simulink model "psbmachinesR12"  (Simulink 4.00)
settings: Solver=ode15s  SolverMode=SingleTasking  StartTime=0.0  StopTime=5  RelTol=1e-3  AbsTol=1e-3
InitFcn:
  | powericon('psbinitsys',bdroot);
undefined symbols (not defined in the file): D1, Delta
libraries: powerlib2 x14, powerlib_extras x5, powerlib11 x2
settings Model: Creator=patrice  LastModifiedBy=pavel  OutputTimes=[0:1/20:10]  LimitDataPoints=off  RTWTemplateMakefile=grt_unix.tmf  ExtModeTrigMode=oneshot  ExtModeArmWhenConnect=off  BlockReductionOpt=off

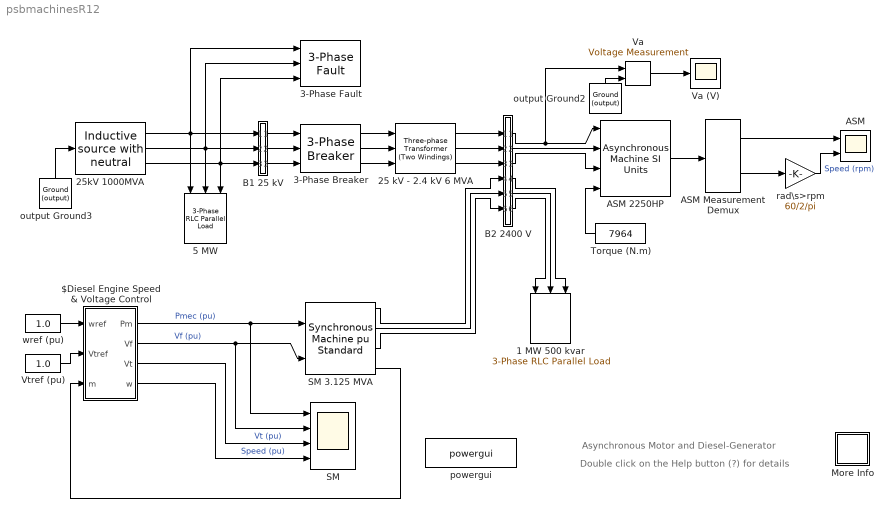
== system psbmachinesR12 ==
  note: Asynchronous Motor and Diesel-Generator
  note: Double click on the Help button (?) for details
  $Diesel Engine Speed & Voltage Control : Subsystem
      settings: RTWFcnNameOpts=Auto  RTWFileNameOpts=Auto
  1 MW 500 kvar : powerlib_extras/Three-Phase Library/3-Phase RLC Parallel Load  Orientation=down  Vpp=2400  fn=60  P3=1e6  QL3=0  QC3=500e3
  25 kV - 2.4 kV 6 MVA : powerlib2/Elements/Three-phase Transformer (Two Windings)  Tag=PoWeRsYsTeMbLoCk  nominal=[ 6e6 , 60 ]  type1=Yg  params1=[ 25e3 , 0.0015 , 0.03]  type2=Delta (D1)  params2=[ 2.4e3 , 0.0015 , 0.03 ]  ynsat=off  rmag=200  lm=200  sat="[ 0,0  ;  0.005,1.2  ;  1.0,1.4 ]"  sif=off  phi0=[ 0.8 , -0.8 , 0.7 ]  mesure=None  PSBOutputType=1111
  25kV 1000MVA : powerlib_extras/Three-Phase Library/Inductive source with neutral  V=25e3/sqrt(3)*sqrt(2)  Phi=0  F=60  R=25^2/1000/10  L=25^2/1000/377
  3-Phase Breaker : powerlib_extras/Three-Phase Library/3-Phase Breaker  init_states=closed  sa=on  sb=on  sc=on  sw_times=[0.2]  Ts=0  comext=off  Ron=0.01  Rp=1e5  Cp=inf  mesure=None
  3-Phase Fault : powerlib_extras/Three-Phase Library/3-Phase Fault  sa=on  sb=on  sc=on  Rdef=0.01  st=on  Rt=0.001  comext=off  sw_status=[1 0]  sw_times=[ 0.1 0.4]  Ts=0  init_statext=[1 1 0]  Rp=inf  Cp=inf  mesure=None
  5 MW : powerlib_extras/Three-Phase Library/3-Phase RLC Parallel Load  Orientation=down  Vpp=25e3  fn=60  P3=5e6  QL3=0  QC3=0
  ASM : Scope  NumInputPorts=2
      settings: TimeRange=0.2  YMin=-7500~1710  YMax=7500~1800  SaveToWorkspace=off  SaveName=ScopeData  DataFormat=Array  MaxDataPoints=5000
  ASM 2250HP : powerlib2/Machines/Asynchronous Machine SI Units  Tag=PoWeRsYsTeMbLoCk  rotType=Squirrel-cage  ctrl=Rotor  x1=[ 2250*746, 2400, 60 ]  x2=[ 0.029 0.226/377]  x3=[ 0.022 0.226/377]  x4=13.04/377  x5="[ 63.87 0  2 ]"  x6=[1 0 0 0 0 0 0 0]  PSBOutputType=1110  iounits=1
  ASM Measurement Demux : powerlib11/Machines/ASM Measurement Demux  a=off  b=off  c=off  d=off  e=on  f=off  g=off  h=off  i=on  j=off  k=off
  B1 25 kV : Subsystem
      settings: RTWFcnNameOpts=Auto  RTWFileNameOpts=Auto
      mask Display: disp('')
  B2 2400 V : Subsystem
      settings: RTWFcnNameOpts=Auto  RTWFileNameOpts=Auto
      mask Display: disp('')
  More Info : Subsystem
      settings: RTWFcnNameOpts=Auto  RTWFileNameOpts=Auto
      mask Display: disp('?')
  SM : Scope  NumInputPorts=4
      settings: TimeRange=0.2  YMin=0.8025~0~0.9825~1.00115  YMax=0.8175~2.75~1.005~1.00155  SaveName=Pmec_SM  DataFormat=Structure  MaxDataPoints=5000  Decimation=10
  SM 3.125 MVA : powerlib2/Machines/Synchronous Machine pu Standard  Tag=PoWeRsYsTeMbLoCk  rotorType=Salient-pole  x1="[ 3.125e6  2400  60 ]"  x2b=[ 31 32 33 34 35 36 37 ]  x2=[ 1.56, 0.296, 0.177, 1.06, 0.177, 0.052 ]  dAxisT=Short-circuit  qAxisT=Open-circuit  x3a=[]  x3b=[]  x3c=[]  x3d=[]  x3=[ 3.7, 0.05, 0.05 ]  x3e=[]  x3f=[]  x3g=[]  x4=0.0036  x5="[ 1.07  0  2 ]"  x6=[0 0 0 0 0 0 0 0 1]  x7=off  x8=[0.211 0.418 1.0 1.72 3.35 ; 0.25 0.50 1.0 1.2 1.4]  PSBOutputType=1110  iounits=0.5
  Torque (N.m) : Constant  Orientation=left  Value=7964
  Va : powerlib2/Measurements/Voltage Measurement  Tag=PoWeRsYsTeMmEaSuReMeNt  PSBOutputType=0  PSBequivalent=0
  Va (V) : Scope
      settings: TickLabels=on  TimeRange=0.2  YMin=-2000  YMax=2000  SaveToWorkspace=off  SaveName=ScopeData  DataFormat=Array  MaxDataPoints=5000
  Vtref (pu) : Constant  Value=1.0
  output Ground2 : powerlib2/Connectors/Ground (output)  Tag=PoWeRsYsTeMbLoCk  Orientation=up  PSBOutputType=1
  output Ground3 : powerlib2/Connectors/Ground (output)  Tag=PoWeRsYsTeMbLoCk  Orientation=up  PSBOutputType=1
  powergui : powerlib2/powergui  matfilesaved=off  Frange=logspace(0,3,50)  Ylog=off  Xlog=off  save=off  variable=ZData  display=off
  rad\s>rpm : Gain  Gain=60/2/pi  Multiplication=Element-wise(K.*u)  SaturateOnIntegerOverflow=on
  wref (pu) : Constant  Value=1.0
  wires:
  25kV 1000MVA/3 -> B1 25 kV/3(C1), 5 MW/3, 3-Phase Fault/3
  25kV 1000MVA/2 -> B1 25 kV/2(B1), 5 MW/2, 3-Phase Fault/2
  25kV 1000MVA/1 -> B1 25 kV/1(A1), 5 MW/1, 3-Phase Fault/1
  output Ground3/1 -> 25kV 1000MVA/1
  B1 25 kV/3(C2) -> 3-Phase Breaker/3
  B1 25 kV/2(B2) -> 3-Phase Breaker/2
  B1 25 kV/1(A2) -> 3-Phase Breaker/1
  3-Phase Breaker/1 -> 25 kV - 2.4 kV 6 MVA/1
  wref (pu)/1 -> $Diesel Engine Speed & Voltage Control/1(wref)
  SM 3.125 MVA/4 -> $Diesel Engine Speed & Voltage Control/3(m)
  Vtref (pu)/1 -> $Diesel Engine Speed & Voltage Control/2(Vtref)
  3-Phase Breaker/3 -> 25 kV - 2.4 kV 6 MVA/3
  3-Phase Breaker/2 -> 25 kV - 2.4 kV 6 MVA/2
  25 kV - 2.4 kV 6 MVA/3 -> B2 2400 V/3(C1)
  25 kV - 2.4 kV 6 MVA/2 -> B2 2400 V/2(B1)
  25 kV - 2.4 kV 6 MVA/1 -> B2 2400 V/1(A1`)
  SM 3.125 MVA/1 -> B2 2400 V/4(A2)
  SM 3.125 MVA/2 -> B2 2400 V/5(B2)
  SM 3.125 MVA/3 -> B2 2400 V/6(C2)
  B2 2400 V/1(A3) -> ASM 2250HP/1, Va/1
  Torque (N.m)/1 -> ASM 2250HP/4
  ASM 2250HP/1 -> ASM Measurement Demux/1
  B2 2400 V/4(A4) -> 1 MW 500 kvar/3
  B2 2400 V/5(B4) -> 1 MW 500 kvar/2
  B2 2400 V/6(C4) -> 1 MW 500 kvar/1
  B2 2400 V/2(B3) -> ASM 2250HP/2
  B2 2400 V/3(C3) -> ASM 2250HP/3
  Va/1 -> Va (V)/1
  output Ground2/1 -> Va/2
  $Diesel Engine Speed & Voltage Control/1(Pm) -> SM 3.125 MVA/1, SM/1  "Pmec (pu)"
  $Diesel Engine Speed & Voltage Control/2(Vf) -> SM 3.125 MVA/2, SM/2  "Vf (pu)"
  $Diesel Engine Speed & Voltage Control/3(Vt) -> SM/3  "Vt (pu)"
  $Diesel Engine Speed & Voltage Control/4(w) -> SM/4  "Speed (pu)"
  ASM Measurement Demux/2 -> rad\s>rpm/1
  ASM Measurement Demux/1 -> ASM/1
  rad\s>rpm/1 -> ASM/2  "Speed (rpm)"

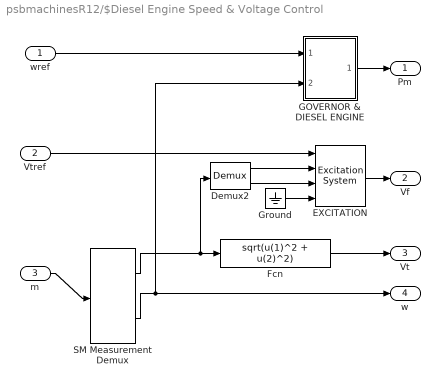
== system psbmachinesR12/$Diesel Engine Speed & Voltage Control ==
  wref : Inport  Port=1
  Vtref : Inport  Port=2
  m : Inport  Port=3
  Demux2 : Demux  Outputs=2  BusSelectionMode=off
  EXCITATION : powerlib2/Machines/Excitation System  tr=20e-3  reg=[ 200, 0.02 ]  exc=[ 1, 0 ]  tgr=[ 0, 0 ]  damp=[ 0.001, 0.1 ]  sat=[ 0, 0 ]  lim=[ 0, 6, 0 ]  v0="[1.0  1.182]"
  Fcn : Fcn  Expr=sqrt(u(1)^2 + u(2)^2)
  GOVERNOR & DIESEL ENGINE : Subsystem  mask(Diesel Engine & Governor){K=40, Tr=[0.01 0.02 0.2], Ta=[0.25 0.009 0.0384], Tlim=[0 1.1], Td=0.024, Pm0=0.1601}
      mask prompts: K "Regulator gain K:"; Tr "Regulator time constants [T1 T2 T3 ] (s) :"; Ta "Actuator time constants [T4 T5 T6] (s) :"; Tlim "Torque limits [Tmin Tmax] (pu) :"; Td "Engine time delay Td (s) :"; Pm0 "Initial value of mechanical power  Pm0 (pu) :"
      mask help:
      | This block implements a diesel engine and governor system:
      | 1st and 2nd inputs: Desired and actual speed (pu)
      | Output: Diesel engine mechanical power.Motor inertia should be combined with generator.
      | Controller transfer function:
      |      Hc=K.(1+T3.s)/(1+T1.s+T1.T2.s^2)
      | Actuator transfer function :
      |      Ha= (1+T4.s) / [ (s (1+T5.s)(1+T6.s) ]
      | Motor :
      |      Time delay Td
      |
      | (See reference in Tutorial Session 5)
      settings: RTWFcnNameOpts=Auto  RTWFileNameOpts=Auto
  Ground : Ground
  SM Measurement Demux : powerlib11/Machines/SM Measurement Demux  a=off  b=off  c=off  d=off  e=off  f=on  g=off  h=on  i=off  j=off
  Pm : Outport  Port=1  InitialOutput=0
  Vf : Outport  Port=2  InitialOutput=0
  Vt : Outport  Port=3  InitialOutput=0
  w : Outport  Port=4  InitialOutput=0
  wires:
  Fcn/1 -> Vt/1
  SM Measurement Demux/1 -> Fcn/1, Demux2/1
  Demux2/1 -> EXCITATION/2
  Vtref/1 -> EXCITATION/1
  GOVERNOR & DIESEL ENGINE/1(Pmec (pu)) -> Pm/1
  EXCITATION/1 -> Vf/1
  Demux2/2 -> EXCITATION/3
  wref/1 -> GOVERNOR & DIESEL ENGINE/1(wref (pu))
  SM Measurement Demux/2 -> w/1, GOVERNOR & DIESEL ENGINE/2(w (pu))
  m/1 -> SM Measurement Demux/1
  Ground/1 -> EXCITATION/4

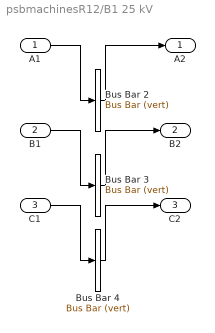
== system psbmachinesR12/B1 25 kV ==
  A1 : Inport  Port=1
  B1 : Inport  Port=2
  C1 : Inport  Port=3
  Bus Bar 2 : powerlib2/Connectors/Bus Bar (vert)  Tag=PoWeRsYsTeMbLoCk  entrees=1  sorties=1  PSBOutputType=11111111111111111111111111111111111111111111111111111111111111111111111111111111111111111
  Bus Bar 3 : powerlib2/Connectors/Bus Bar (vert)  Tag=PoWeRsYsTeMbLoCk  entrees=1  sorties=1  PSBOutputType=11111111111111111111111111111111111111111111111111111111111111111111111111111111111111111
  Bus Bar 4 : powerlib2/Connectors/Bus Bar (vert)  Tag=PoWeRsYsTeMbLoCk  entrees=1  sorties=1  PSBOutputType=11111111111111111111111111111111111111111111111111111111111111111111111111111111111111111
  A2 : Outport  Port=1  InitialOutput=0
  B2 : Outport  Port=2  InitialOutput=0
  C2 : Outport  Port=3  InitialOutput=0
  wires:
  A1/1 -> Bus Bar 2/1
  Bus Bar 2/1 -> A2/1
  B1/1 -> Bus Bar 3/1
  Bus Bar 3/1 -> B2/1
  C1/1 -> Bus Bar 4/1
  Bus Bar 4/1 -> C2/1

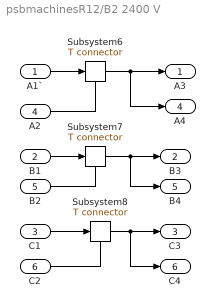
== system psbmachinesR12/B2 2400 V ==
  A1` : Inport  Port=1
  B1 : Inport  Port=2
  C1 : Inport  Port=3
  A2 : Inport  Port=4
  B2 : Inport  Port=5
  C2 : Inport  Port=6
  Subsystem6 : powerlib2/Connectors/T connector  Tag=PoWeRsYsTeMbLoCk  PSBOutputType=1
  Subsystem7 : powerlib2/Connectors/T connector  Tag=PoWeRsYsTeMbLoCk  PSBOutputType=1
  Subsystem8 : powerlib2/Connectors/T connector  Tag=PoWeRsYsTeMbLoCk  PSBOutputType=1
  A3 : Outport  Port=1  InitialOutput=0
  B3 : Outport  Port=2  InitialOutput=0
  C3 : Outport  Port=3  InitialOutput=0
  A4 : Outport  Port=4  InitialOutput=0
  B4 : Outport  Port=5  InitialOutput=0
  C4 : Outport  Port=6  InitialOutput=0
  wires:
  Subsystem8/1 -> C4/1, C3/1
  Subsystem7/1 -> B4/1, B3/1
  Subsystem6/1 -> A4/1, A3/1
  C2/1 -> Subsystem8/Enable
  A2/1 -> Subsystem6/Enable
  B2/1 -> Subsystem7/Enable
  B1/1 -> Subsystem7/1
  C1/1 -> Subsystem8/1
  A1`/1 -> Subsystem6/1

== system psbmachinesR12/More Info ==
  note: Observe that during the fault the terminal voltage drops to about 0.2 pu and the excitation voltage hits the  limit of 6 pu. After fault clearing and islanding
      |  the SM  mechanical power  increases from its initial value of 0.16 pu to the final value of 0.80 pu required by the resistive and motor load (2.49 MW) . After 3 seconds,
      |  the terminal voltage stabilizes at 1 pu. The motor speed decreases transiently from 1789 rpm to 1624 rpm, then it recovers close to its normal value after 2 seconds.
      |
      | If you  increase the fault duration to 12 cycles by changing the breaker opening time to 0.3s, you will notice that the system collapses.
      |  The ASM speed slows down to zero after 2 seconds.
  note: 3
  note: 1
  note: Demonstration
  note: Circuit Description
  note: This demonstration illustrates fault and islanding of an induction motor/diesel-generator system.
      | It also demonstrates the Machine Load Flow option of the PowerGUI .
      | ( See Tutorial Session 5)
  note: A plant consisting of a resistive and motor load (ASM) is fed at 2400 V from a distibution 25 kV network through a 6 MVA 25/2.kV Wye-Delta transformer and from an
      | emergency synchronous generator/ diesel engine unit (SM). The 25 kV network is modelled by a simple R-L equivalent source (short-circuit level 1000 MVA) and a 5 MW load.
      |  The  asynchronous motor is  rated 2250 HP, 2.4 kV and the synchronous machine is rated 3.125 MVA, 2.4kV. The SM excitation is performed by the standard
      |  excitation block provided with Powerlib. The diesel engine and governor system are modelled by a SIMULINK block (See tutorial, session 5 in the user`s manual).
      | Initially, the motor develops a mechanical power of 2000 HP (1.49 MW) and the diesel generator provides 500 kW (0.16 pu) of active power.
      | The generator controls the 2400V bus B2 voltage at 1pu and generates 500kW (0.16 pu) of active power.  At t=0.1 s, a three-phase to ground
      |  fault occurs on the 25 kV system, causing opening of the 25kV circuit breaker at t=0.2 s .
      |
      | The demonstration illustrates the mecanical and electrical transients following the fault and islanding of the Motor/Generator system.
  note: Open the 4  scopes displaying the terminal voltge, field voltage, mechanical power and speed of the synchronous machine as well as
      | the scope displaying the asynchronous motor speed. Start the simulation.
  note: Start Simulation. If the SM and ASM initial conditions are not properly set you  will  observe that the voltage and currents Machine do not start in steady state.
      |  Stop the simulation.
  note: 2
  note: In order to start the simulation in steady-state you must initialize the synchronous machine and the asynchronous motor for the desired load flow.
      | Open the  POWERGUI and select "Load Flow & Machine initialization" in the Tools menu. The machine "Bus type" should be already initialized as "PV generator",
      |  indicating that  the load flow will be performed with the machine controlling its active power and terminal voltage. Specify the desired values by entering
      |  the following parameters : U AB (Vrms) = 2400;  P (wattts) =500e3. Specify also the ASM mechanical power by entering Pmec (Watts)= 2000*746.
      |  Then press the "Execute Load Flow" button
      | .
      |  Once the load flow is solved the phasors of AB and BC machine voltages and currents flowing in phases A and B are updated.
      |  The SM reactive power,  mechanical power and  field voltage are displayed : Q =315 kvar; Pmec=500 kW (0.1601 pu) ; field voltage Ef=1.182 pu;
      |  The active and reactive powers absorbed by the motor,  slip and torque are also displayed.
  note: As the diesel engine governor and SM excitation system contain several states, they should also be initialized according to the values calculated by the load flow.
      |  Open the GOVERNOR block in the Diesel Engine subsystem. The initial mechanical power has been set to 0.1601 pu in the GOVERNOR.
      | Now open the EXCITATION block. The initial terminal voltage and field voltage have been set respectively to 1.0 and 1.182 pu.
  note: 4
  note: G. Sybille ; Hydro-Quebec (IREQ)

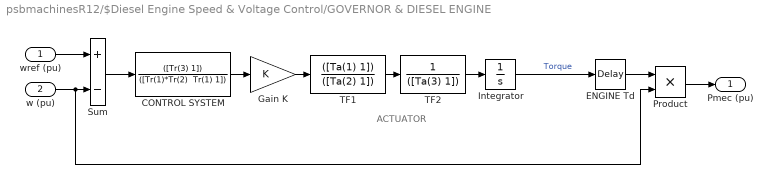
== system psbmachinesR12/$Diesel Engine Speed & Voltage Control/GOVERNOR & DIESEL ENGINE ==
  note: ACTUATOR
  wref (pu) : Inport  Port=1
  w (pu) : Inport  Port=2
  CONTROL SYSTEM : TransferFcn  Numerator=([Tr(3) 1])  Denominator="([Tr(1)*Tr(2)  Tr(1) 1])"  Realization=auto  AbsoluteTolerance=auto
  ENGINE Td : TransportDelay  DelayTime=Td  InitialInput=Pm0  BufferSize=1024  PadeOrder=0
  Gain K : Gain  Gain=K  Multiplication=Element-wise(K.*u)  SaturateOnIntegerOverflow=on
  Integrator : Integrator  ExternalReset=none  InitialConditionSource=internal  InitialCondition=Pm0  LimitOutput=on  UpperSaturationLimit=Tlim(2)  LowerSaturationLimit=Tlim(1)  ShowSaturationPort=off  ShowStatePort=off  AbsoluteTolerance=auto
  Product : Product  Inputs=2  Multiplication=Element-wise(.*)  SaturateOnIntegerOverflow=on
  Sum : Sum  Inputs=+-  SaturateOnIntegerOverflow=on
  TF1 : TransferFcn  Numerator=([Ta(1) 1])  Denominator=([Ta(2) 1])  Realization=auto  AbsoluteTolerance=auto
  TF2 : TransferFcn  Numerator=1  Denominator=([Ta(3) 1])  Realization=auto  AbsoluteTolerance=auto
  Pmec (pu) : Outport  Port=1  InitialOutput=0
  wires:
  Integrator/1 -> ENGINE Td/1  "Torque"
  TF2/1 -> Integrator/1
  Product/1 -> Pmec (pu)/1
  wref (pu)/1 -> Sum/1
  ENGINE Td/1 -> Product/1
  w (pu)/1 -> Sum/2, Product/2
  TF1/1 -> TF2/1
  CONTROL SYSTEM/1 -> Gain K/1
  Sum/1 -> CONTROL SYSTEM/1
  Gain K/1 -> TF1/1
